simulink model "PFC_Plant_2022b_final"  (R2023b)
settings: Solver=FixedStepAuto  StartTime=0.0  StopTime=0.5  FixedStep=1e-5  RelTol=1e-3
undefined symbols (not defined in the file or in its folder): DiscIntNeverNeededParam
libraries: simulink x5, spsMeanLib x4, eeGeneralControl x2, eePowerMeasurement x1, spsTHDLib x1
settings Model: PacingRate=1000  Creator=tuca_v1  LastModifiedBy=Moisa Versatu
settings OptimizationCC: ReuseModelBlockBuffer=off
settings DebuggingCC: UnconnectedInputMsg=warning  UnconnectedOutputMsg=warning  UnconnectedLineMsg=warning
settings ModelReferenceCC: EnableRefExpFcnMdlSchedulingChecks=on
settings RTWCC: DLArmComputeVersion=19.05

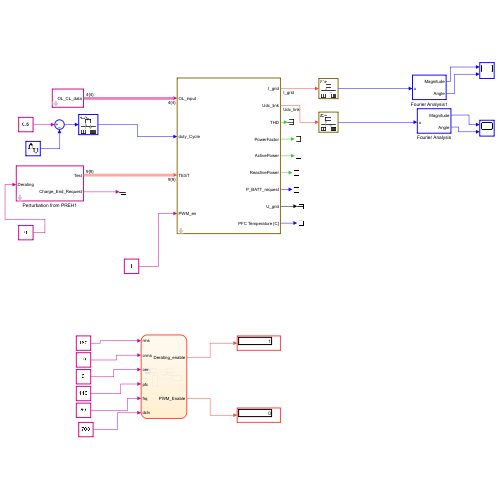
[thumbnail: Simulink's stored preview of the top-level diagram]
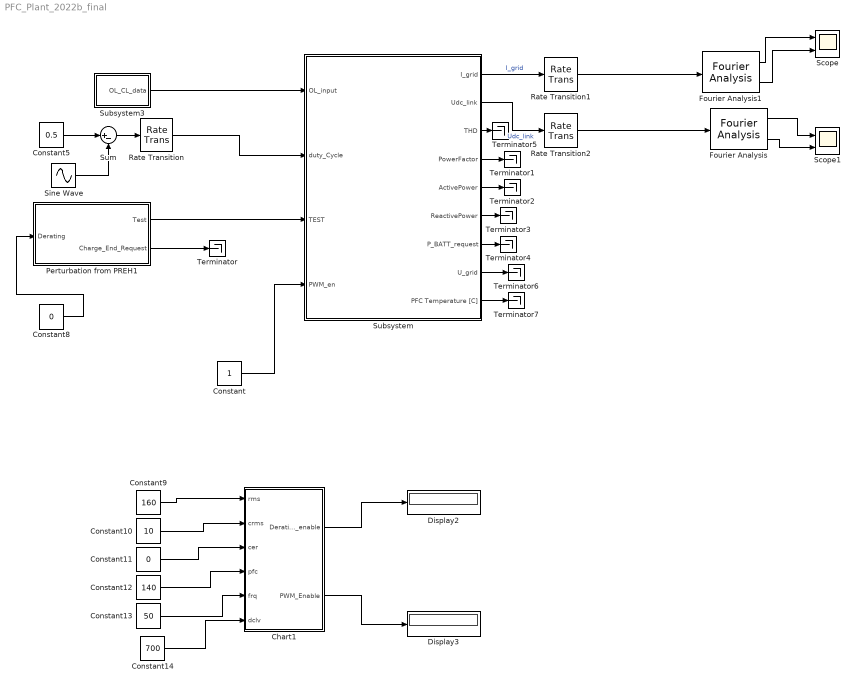
== system PFC_Plant_2022b_final ==
  Chart1 : Stateflow chart  TreatAsAtomicUnit=on
  Constant : Constant
  Constant10 : Constant  Value=10
  Constant11 : Constant  Value=0
  Constant12 : Constant  Value=140
  Constant13 : Constant  Value=50
  Constant14 : Constant  Value=700
  Constant5 : Constant  Value=0.5
  Constant8 : Constant  Value=0
  Constant9 : Constant  Value=160
  Display2 : Display
  Display3 : Display
  Fourier Analysis : eeGeneralControl/Fourier Analysis  f=50  n=[1]  M0=1  Ph0=0  BufferSize=8192  Ts=1e-4
      settings: LibrarySourceBlock=ee_sl_lib/General Control/Fourier Analysis
  Fourier Analysis1 : eeGeneralControl/Fourier Analysis  f=50  n=[1]  M0=1  Ph0=0  BufferSize=8192  Ts=1e-4
      settings: LibrarySourceBlock=ee_sl_lib/General Control/Fourier Analysis
  Perturbation from PREH1 : Subsystem  mask{Overwrite_power=0, Uin_rms=220, F_grid=50, RMS_variation=0, Freq_variation=0, AC_harmonics=0, Charge_End_Request=0, Coolant_mass_flow=0.1, Coolant_temperature=60}
      mask prompts: Charge_End_Request "Charge End Request"
  Rate Transition : RateTransition  OutPortSampleTime=1e-4
  Rate Transition1 : RateTransition  OutPortSampleTime=1e-4
  Rate Transition2 : RateTransition  OutPortSampleTime=1e-4
  Scope : Scope  NumInputPorts=2
  Scope1 : Scope  NumInputPorts=2
  Sine Wave : Sin  Amplitude=0.02  Frequency=2*pi*50  SampleTime=1e-4
  Subsystem : Subsystem  mask{f_grid=50}
      mask init:
      | Ts_thermal = 1e-2;
      | Tc = 1e-5;
  Subsystem3 : Subsystem  mask{DC_AC=0, Uin_rms_OL=220, UDC_link_OL=220, Power_out=0}
      mask prompts: DC_AC "DC_AC enum"
  Sum : Sum  Inputs=|+-
  Terminator{,1..7} (8 alike) : Terminator
  wires:
  Subsystem3/1(OL_CL_data) -> Subsystem/1(OL_input)
  Subsystem/8(U_grid) -> Terminator6/1
  Perturbation from PREH1/1(Test) -> Subsystem/3(TEST)
  Constant5/1 -> Sum/1
  Sine Wave/1 -> Sum/2
  Sum/1 -> Rate Transition/1
  Rate Transition/1 -> Subsystem/2(duty_Cycle)
  Subsystem/2(Udc_link) -> Rate Transition2/1  "Udc_link"
  Subsystem/1(I_grid) -> Rate Transition1/1  "I_grid"
  Rate Transition2/1 -> Fourier Analysis/1
  Constant/1 -> Subsystem/4(PWM_en)
  Constant8/1 -> Perturbation from PREH1/1(Derating)
  Perturbation from PREH1/2(Charge_End_Request) -> Terminator/1
  Subsystem/7(P_BATT_request) -> Terminator4/1
  Subsystem/6(ReactivePower) -> Terminator3/1
  Subsystem/5(ActivePower) -> Terminator2/1
  Subsystem/4(PowerFactor) -> Terminator1/1
  Subsystem/3(THD) -> Terminator5/1
  Subsystem/9(PFC Temperature [C]) -> Terminator7/1
  Rate Transition1/1 -> Fourier Analysis1/1
  Fourier Analysis/1 -> Scope1/1
  Fourier Analysis1/1 -> Scope/1
  Chart1/1(Derating_enable) -> Display2/1
  Constant11/1 -> Chart1/3(cer)
  Constant10/1 -> Chart1/2(crms)
  Constant9/1 -> Chart1/1(rms)
  Constant13/1 -> Chart1/5(frq)
  Constant14/1 -> Chart1/6(dclv)
  Constant12/1 -> Chart1/4(pfc)
  Chart1/2(PWM_Enable) -> Display3/1
  Fourier Analysis1/2 -> Scope/2
  Fourier Analysis/2 -> Scope1/2

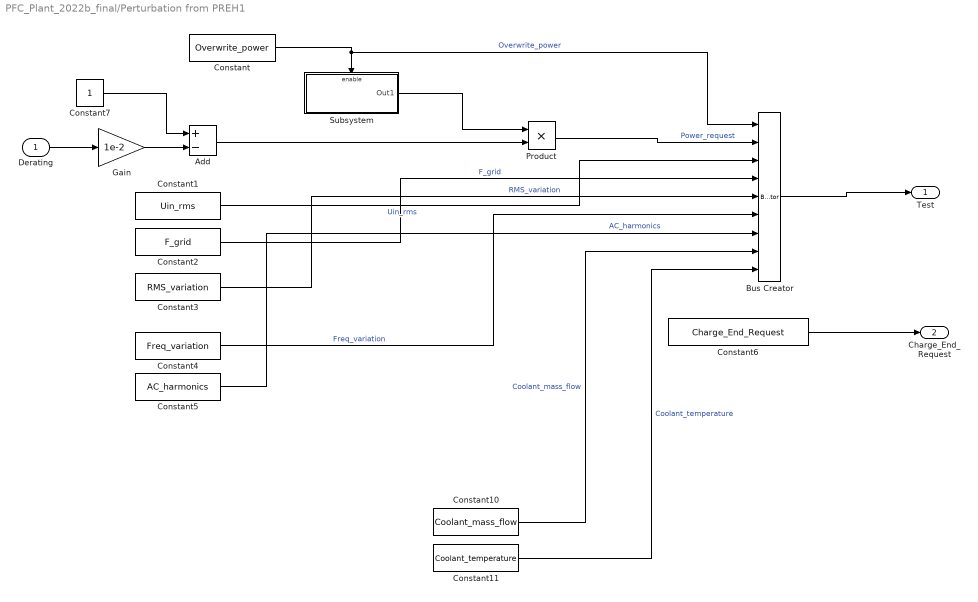
== system PFC_Plant_2022b_final/Perturbation from PREH1 ==
  Derating : Inport
  Add : Sum  Inputs=+-
  Bus Creator : BusCreator  Inputs=9
  Constant : Constant  Value=Overwrite_power
  Constant1 : Constant  Value=Uin_rms
  Constant10 : Constant  Value=Coolant_mass_flow
  Constant11 : Constant  Value=Coolant_temperature
  Constant2 : Constant  Value=F_grid
  Constant3 : Constant  Value=RMS_variation
  Constant4 : Constant  Value=Freq_variation
  Constant5 : Constant  Value=AC_harmonics
  Constant6 : Constant  Value=Charge_End_Request
  Constant7 : Constant
  Gain : Gain  Gain=1e-2
  Product : Product
  Subsystem : Subsystem
  Test : Outport
  Charge_End_Request : Outport  Port=2
  wires:
  Constant/1 -> Bus Creator/1, Subsystem/Enable  "Overwrite_power"
  Bus Creator/1 -> Test/1
  Subsystem/1(Out1) -> Product/1
  Constant1/1 -> Bus Creator/3  "Uin_rms"
  Constant2/1 -> Bus Creator/4  "F_grid"
  Constant3/1 -> Bus Creator/5  "RMS_variation"
  Constant4/1 -> Bus Creator/6  "Freq_variation"
  Constant5/1 -> Bus Creator/7  "AC_harmonics"
  Add/1 -> Product/2
  Product/1 -> Bus Creator/2  "Power_request"
  Constant6/1 -> Charge_End_Request/1
  Gain/1 -> Add/2
  Derating/1 -> Gain/1
  Constant7/1 -> Add/1
  Constant10/1 -> Bus Creator/8  "Coolant_mass_flow"
  Constant11/1 -> Bus Creator/9  "Coolant_temperature"

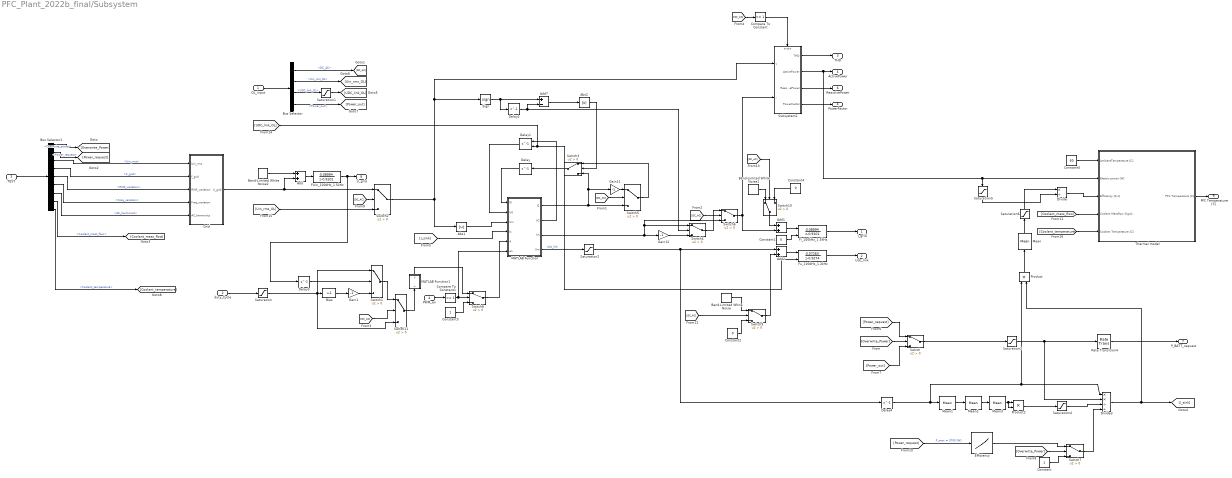
== system PFC_Plant_2022b_final/Subsystem ==
  OL_input : Inport
  duty_Cycle : Inport  Port=2
  TEST : Inport  Port=3
  PWM_en : Inport  Port=4
  Abs1 : Abs  SaturateOnIntegerOverflow=off
  Abs2 : Abs  SaturateOnIntegerOverflow=off
  Add : Sum
  Add1 : Sum
  Add2 : Sum
  Add7 : Sum  Inputs=+-
  Band-Limited White Noise : simulink/Sources/Band-Limited White Noise  Cov=5e-7  Ts=1e-5  seed=[23341]
  Band-Limited White Noise1 : simulink/Sources/Band-Limited White Noise  Cov=5e-9  Ts=1e-5  seed=[23342]
  Band-Limited White Noise2 : simulink/Sources/Band-Limited White Noise  Cov=5e-7  Ts=1e-5  seed=[23342]
  Bias : Bias  Bias=-1  SaturateOnIntegerOverflow=off
  Bus Selector : BusSelector  OutputSignals=DC_AC,Uin_rms_OL,UDC_link_OL,Power_out
  Bus Selector1 : BusSelector  OutputSignals=Overwrite_power,Power_request,Uin_rms,F_grid,RMS_variation,Freq_variation,AC_harmonics,Coolant_mass_flow,Coolant_temperature
  Compare To Constant : simulink/Logic and Bit Operations/Compare To Constant  relop===  const=1  OutDataTypeStr=boolean
  Compare To Constant1 : simulink/Logic and Bit Operations/Compare To Constant  relop===  const=1  OutDataTypeStr=boolean
  Constant : Constant
  Constant1 : Constant  Value=0
  Constant2 : Constant  Value=0
  Constant3 : Constant
  Constant4 : Constant  Value=0
  Constant5 : Constant  Value=60
  Delay : Delay  DelayLength=1  SampleTime=1e-5
  Delay1 : Delay  DelayLength=1  InitialConditionSource=Input port  SampleTime=1e-5
      settings: InputPortMap=u0,p4
  Delay2 : Delay  DelayLength=1  SampleTime=1e-5
  Delay3 : Delay  DelayLength=1  SampleTime=Tc
  Delay4 : Delay  DelayLength=1  SampleTime=Tc
  Divide : Product  Inputs=*/
  Divide3 : Product  Inputs=**//
  Efficiency : Lookup_n-D  NumberOfTableDimensions=1  BreakpointsForDimension1=[500 1000 1500 2000 2500 3000 3500 5000 7000 9000 11100]/3  Table="[0.85 0.92 0.95  0.97  0.975 0.97 0.967 0.963 0.96 0.959 0.955]"  ExtrapMethod=Clip  UseLastTableValue=on  InternalRulePriority=Speed  RndMeth=Simplest
  FUin_100kHz_1.5kHz : DiscreteTransferFcn  Numerator=[0.08994]  Denominator=[1 -0.9101]  SampleTime=Tc
  Fi_100kHz_1.5kHz : DiscreteTransferFcn  Numerator=[0.08994]  Denominator=[1 -0.9101]  InitialStatesSource=Input port  SampleTime=Tc
      settings: InputPortMap=u0,p5
  Fu_100kHz_1.2kHz : DiscreteTransferFcn  Numerator=[0.07263]  Denominator=[1 -0.9274]  InitialStatesSource=Input port  SampleTime=Tc
      settings: InputPortMap=u0,p5
  Gain1 : Gain  Gain=-1
  Gain11 : Gain  Gain=-1
  Gain12 : Gain  Gain=-1
  Grid : Subsystem
  MATLAB Function : MATLAB Function  TreatAsAtomicUnit=on
  MATLAB Function1 : MATLAB Function  TreatAsAtomicUnit=on
  Mean : spsMeanLib/Mean  Freq=5  Vinit=0  Ts=Tc
  Mean1 : spsMeanLib/Mean  Freq=2*f_grid  Vinit=0  Ts=Tc
  Mean2 : spsMeanLib/Mean  Freq=2*f_grid  Vinit=0  Ts=Tc
  Mean3 : spsMeanLib/Mean  Freq=2*f_grid  Vinit=0  Ts=Tc
  Product : Product
  Product2 : Product
  Rate Transition4 : RateTransition  OutPortSampleTime=1e-2
  Saturation : Saturate  UpperLimit=0.998  LowerLimit=0.002
  Saturation1 : Saturate  UpperLimit=inf  LowerLimit=1e-4
  Saturation2 : Saturate  UpperLimit=inf  LowerLimit=1e-4
  Saturation3 : Saturate  UpperLimit=1e3  LowerLimit=0
  Saturation4 : Saturate  UpperLimit=inf  LowerLimit=1e-4
  Saturation5 : Saturate  UpperLimit=1e4  LowerLimit=1
  Saturation6 : Saturate  UpperLimit=1e4  LowerLimit=1
  Sign : Signum
  Subsystem1 : Subsystem
  Switch{,1..11} (12 alike) : Switch  Criteria=u2 > Threshold  SaturateOnIntegerOverflow=off  InputSameDT=off
  Thermal model : Subsystem
  I_grid : Outport
  Udc_link : Outport  Port=2
  THD : Outport  Port=3
  PowerFactor : Outport  Port=4
  ActivePower : Outport  Port=5
  ReactivePower : Outport  Port=6
  P_BATT_request : Outport  Port=7
  U_grid : Outport  Port=8
  PFC Temperature [C] : Outport  Port=9
  wires:
  MATLAB Function/1(I2) -> Switch3/3, Gain11/1, Switch5/3
  Gain12/1 -> Switch4/3
  [UDC_link_OL] -> Delay1/2, Fu_100kHz_1.2kHz/2
  [I_sink] -> MATLAB Function/4(Is)
  Abs2/1 -> Switch3/2
  Add7/1 -> Abs2/1
  Delay1/1 -> MATLAB Function/2(U0)
  Switch3/1 -> Delay/1
  Abs1/1 -> MATLAB Function/3(Uin)
  duty_Cycle/1 -> Saturation/1
  Sign/1 -> Delay2/1, Add7/1
  Switch5/1 -> Switch3/1
  Delay2/1 -> Switch4/2, Add7/2
  MATLAB Function/2(U2) -> Delay1/1
  MATLAB Function/3(Im) -> Gain12/1, Switch4/1, Switch6/3
  Switch6/1 -> Subsystem1/2(i), Add1/2
  Saturation/1 -> Switch11/3, Switch1/1, Bias/1
  Bias/1 -> Gain1/1
  Add1/1 -> Fi_100kHz_1.5kHz/1
  Add2/1 -> Fu_100kHz_1.2kHz/1
  Band-Limited White Noise1/1 -> Switch10/1
  Fi_100kHz_1.5kHz/1 -> I_grid/1
  Fu_100kHz_1.2kHz/1 -> Udc_link/1
  Switch2/1 -> Subsystem1/1(v), Sign/1, Abs1/1
  [Uin_rms_OL] -> Switch2/3
  Gain11/1 -> Switch5/1
  [DC_AC] -> Switch5/2
  [DC_AC] -> Switch6/2
  Switch4/1 -> Switch6/1
  Subsystem1/1(THD) -> THD/1
  Subsystem1/2(ActivePower) -> Thermal model/2(Electric power [W]), Saturation5/1, ActivePower/1
  Subsystem1/3(ReactivePower) -> ReactivePower/1
  Subsystem1/4(PowerFactor) -> PowerFactor/1
  [DC_AC] -> Compare To Constant/1
  Constant1/1 -> Fi_100kHz_1.5kHz/2
  TEST/1 -> Bus Selector1/1
  Switch/1 -> Saturation3/1
  MATLAB Function/4(Um) -> Saturation2/1  "Udc_link"
  Mean1/1 -> Mean2/1
  Rate Transition4/1 -> P_BATT_request/1
  Mean2/1 -> Mean3/1
  Band-Limited White Noise/1 -> Switch9/1
  Switch10/1 -> Add1/1
  [DC_AC] -> Switch2/2
  Mean3/1 -> Product2/2, Product2/1
  Product2/1 -> Saturation4/1
  Saturation3/1 -> Divide3/2, Rate Transition4/1
  Delay4/1 -> Divide3/1, Product/1, Mean1/1
  Compare To Constant/1 -> Subsystem1/Enable
  OL_input/1 -> Bus Selector/1
  Bus Selector/1 -> [DC_AC]  "<DC_AC>"
  Bus Selector/2 -> [Uin_rms_OL]  "<Uin_rms_OL>"
  Bus Selector/3 -> Saturation1/1  "<UDC_link_OL>"
  [DC_AC] -> Switch9/2
  Switch9/1 -> Add2/2
  Constant2/1 -> Switch9/3
  [DC_AC] -> Switch10/2
  Constant4/1 -> Switch10/3
  Grid/1(U_grid) -> Switch2/1, Add/2
  Gain1/1 -> Switch1/3
  Switch11/1 -> MATLAB Function1/1(u)
  Delay3/1 -> Switch1/2
  FUin_100kHz_1.5kHz/1 -> Delay3/1, U_grid/1
  Add/1 -> FUin_100kHz_1.5kHz/1
  Band-Limited White Noise2/1 -> Add/1
  Divide3/1 -> [I_sink], Product/2
  Switch8/1 -> MATLAB Function/5(d)
  Switch1/1 -> Switch11/1
  [DC_AC] -> Switch11/2
  Bus Selector1/1 -> [Overwrite_Power]  "<Overwrite_power>"
  [Overwrite_Power] -> Switch/2
  Bus Selector1/2 -> [Power_request]  "<Power_request>"
  [Power_request] -> Switch/1
  Bus Selector/4 -> [Power_out]  "<Power_out>"
  [Power_out] -> Switch/3
  Switch7/1 -> Divide3/4
  [Overwrite_Power] -> Switch7/2
  Efficiency/1 -> Switch7/1
  Constant/1 -> Switch7/3
  [Power_request] -> Efficiency/1  "P_max = 3700 [W]"
  Bus Selector1/3 -> Grid/1(Uin_rms)  "<Uin_rms>"
  Bus Selector1/4 -> Grid/2(f_grid)  "<F_grid>"
  Bus Selector1/5 -> Grid/3(RMS_variation)  "<RMS_variation>"
  Bus Selector1/6 -> Grid/4(Freq_variation)  "<Freq_variation>"
  Bus Selector1/7 -> Grid/5(AC_harmonics)  "<AC_harmonics>"
  Saturation2/1 -> Add2/1, Delay4/1
  Saturation1/1 -> [UDC_link_OL]
  Saturation4/1 -> Divide3/3
  PWM_en/1 -> Compare To Constant1/1
  Compare To Constant1/1 -> Switch8/2, MATLAB Function/6(en)
  MATLAB Function1/1(y) -> Switch8/1
  Constant3/1 -> Switch8/3
  Delay/1 -> MATLAB Function/1(I0)
  Product/1 -> Mean/1
  Mean/1 -> Saturation6/1
  Divide/1 -> Thermal model/3(Efficiency [0-1])
  Constant5/1 -> Thermal model/1(AmbientTemperature [C])
  [Coolant_temperature] -> Thermal model/5(Coolant Temperature [C])
  [Coolant_mass_flow] -> Thermal model/4(Coolant Massflow [kg/s])
  Thermal model/1(PFC Temperature [C]) -> PFC Temperature [C]/1
  Saturation5/1 -> Divide/2
  Saturation6/1 -> Divide/1
  Bus Selector1/8 -> [Coolant_mass_flow]  "<Coolant_mass_flow>"
  Bus Selector1/9 -> [Coolant_temperature]  "<Coolant_temperature>"

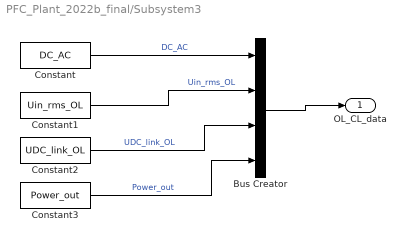
== system PFC_Plant_2022b_final/Subsystem3 ==
  Bus Creator : BusCreator  Inputs=4
  Constant : Constant  Value=DC_AC
  Constant1 : Constant  Value=Uin_rms_OL
  Constant2 : Constant  Value=UDC_link_OL
  Constant3 : Constant  Value=Power_out
  OL_CL_data : Outport
  wires:
  Bus Creator/1 -> OL_CL_data/1
  Constant/1 -> Bus Creator/1  "DC_AC"
  Constant1/1 -> Bus Creator/2  "Uin_rms_OL"
  Constant2/1 -> Bus Creator/3  "UDC_link_OL"
  Constant3/1 -> Bus Creator/4  "Power_out"

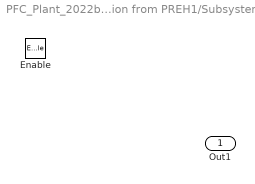
== system PFC_Plant_2022b_final/Perturbation from PREH1/Subsystem ==
  Enable : EnablePort
  Out1 : Outport

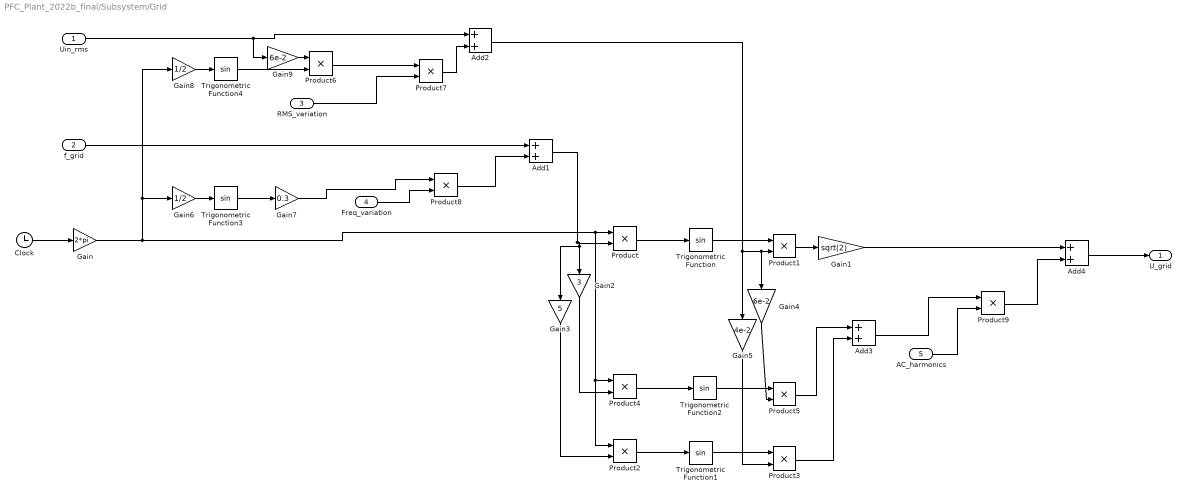
== system PFC_Plant_2022b_final/Subsystem/Grid ==
  Uin_rms : Inport
  f_grid : Inport  Port=2
  RMS_variation : Inport  Port=3
  Freq_variation : Inport  Port=4
  AC_harmonics : Inport  Port=5
  Add1 : Sum
  Add2 : Sum
  Add3 : Sum  Inputs=2
  Add4 : Sum  Inputs=2
  Clock : Clock
  Gain : Gain  Gain=2*pi
  Gain1 : Gain  Gain=sqrt(2)
  Gain2 : Gain  Gain=3
  Gain3 : Gain  Gain=5
  Gain4 : Gain  Gain=6e-2
  Gain5 : Gain  Gain=4e-2
  Gain6 : Gain  Gain=1/2
  Gain7 : Gain  Gain=0.3
  Gain8 : Gain  Gain=1/2
  Gain9 : Gain  Gain=6e-2
  Product{,1..9} (10 alike) : Product
  Trigonometric Function{,1..4} (5 alike) : Trigonometry
  U_grid : Outport
  wires:
  Clock/1 -> Gain/1
  Gain/1 -> Gain8/1, Gain6/1, Product4/1, Product2/1, Product/1
  Product/1 -> Trigonometric Function/1
  Trigonometric Function/1 -> Product1/1
  Product1/1 -> Gain1/1
  Gain1/1 -> Add4/1
  Add1/1 -> Gain3/1, Gain2/1, Product/2
  Product2/1 -> Trigonometric Function1/1
  Trigonometric Function1/1 -> Product3/1
  Add2/1 -> Gain5/1, Gain4/1, Product1/2
  Product3/1 -> Add3/2
  Add4/1 -> U_grid/1
  Trigonometric Function2/1 -> Product5/1
  Product4/1 -> Trigonometric Function2/1
  Product5/1 -> Add3/1
  Gain2/1 -> Product4/2
  Gain3/1 -> Product2/2
  Gain4/1 -> Product5/2
  Gain5/1 -> Product3/2
  f_grid/1 -> Add1/1
  Trigonometric Function3/1 -> Gain7/1
  Gain6/1 -> Trigonometric Function3/1
  Gain7/1 -> Product8/1
  Uin_rms/1 -> Gain9/1, Add2/1
  Gain8/1 -> Trigonometric Function4/1
  Trigonometric Function4/1 -> Product6/2
  Product6/1 -> Product7/1
  Gain9/1 -> Product6/1
  Product7/1 -> Add2/2
  Product8/1 -> Add1/2
  Add3/1 -> Product9/1
  Product9/1 -> Add4/2
  RMS_variation/1 -> Product7/2
  Freq_variation/1 -> Product8/2
  AC_harmonics/1 -> Product9/2

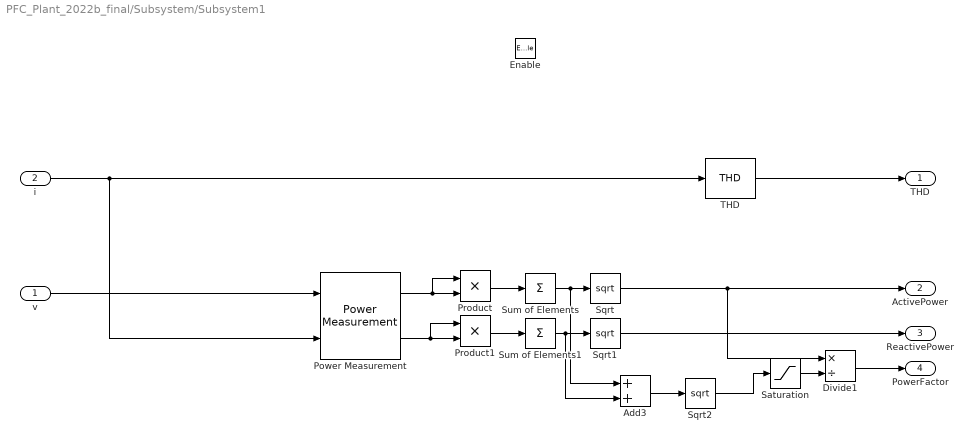
== system PFC_Plant_2022b_final/Subsystem/Subsystem1 ==
  v : Inport
  i : Inport  Port=2
  Enable : EnablePort
  Add3 : Sum
  Divide1 : Product  Inputs=*/
  Power Measurement : eePowerMeasurement/Power Measurement  LabelModeActiveChoice=Discrete  F=f_grid  K=[0 1 2 3 5 7 9 11 13]  Ts=1/2e4
  Product : Product
  Product1 : Product
  Saturation : Saturate  UpperLimit=inf  LowerLimit=1e-4
  Sqrt : Sqrt
  Sqrt1 : Sqrt
  Sqrt2 : Sqrt
  Sum of Elements : Sum  Inputs=+
  Sum of Elements1 : Sum  Inputs=+
  "THD " : spsTHDLib/THD  Freq=f_grid  Ts=1/2e4
  THD : Outport
  ActivePower : Outport  Port=2
  ReactivePower : Outport  Port=3
  PowerFactor : Outport  Port=4
  wires:
  Sqrt/1 -> ActivePower/1, Divide1/1
  Add3/1 -> Sqrt2/1
  Power Measurement/2 -> Product1/1, Product1/2
  "THD "/1 -> THD/1
  Power Measurement/1 -> Product/1, Product/2
  Sum of Elements1/1 -> Add3/2, Sqrt1/1
  Product/1 -> Sum of Elements/1
  i/1 -> Power Measurement/2, "THD "/1
  Sqrt2/1 -> Saturation/1
  Product1/1 -> Sum of Elements1/1
  Sum of Elements/1 -> Add3/1, Sqrt/1
  Sqrt1/1 -> ReactivePower/1
  Divide1/1 -> PowerFactor/1
  v/1 -> Power Measurement/1
  Saturation/1 -> Divide1/2

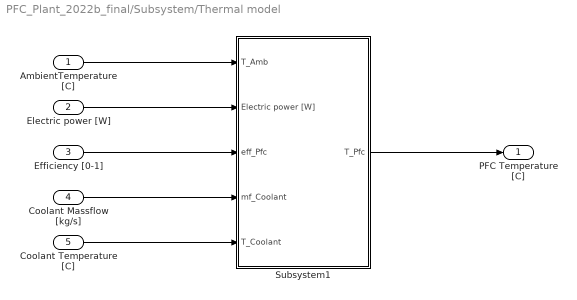
== system PFC_Plant_2022b_final/Subsystem/Thermal model ==
  AmbientTemperature [C] : Inport
  Electric power [W] : Inport  Port=2
  Efficiency [0-1] : Inport  Port=3
  Coolant Massflow [kg/s] : Inport  Port=4
  Coolant Temperature [C] : Inport  Port=5
  Subsystem1 : Subsystem
  PFC Temperature [C] : Outport
  wires:
  Subsystem1/1(T_Pfc) -> PFC Temperature [C]/1
  AmbientTemperature [C]/1 -> Subsystem1/1(T_Amb)
  Coolant Massflow [kg/s]/1 -> Subsystem1/4(mf_Coolant)
  Coolant Temperature [C]/1 -> Subsystem1/5(T_Coolant)
  Electric power [W]/1 -> Subsystem1/2(Electric power [W])
  Efficiency [0-1]/1 -> Subsystem1/3(eff_Pfc)

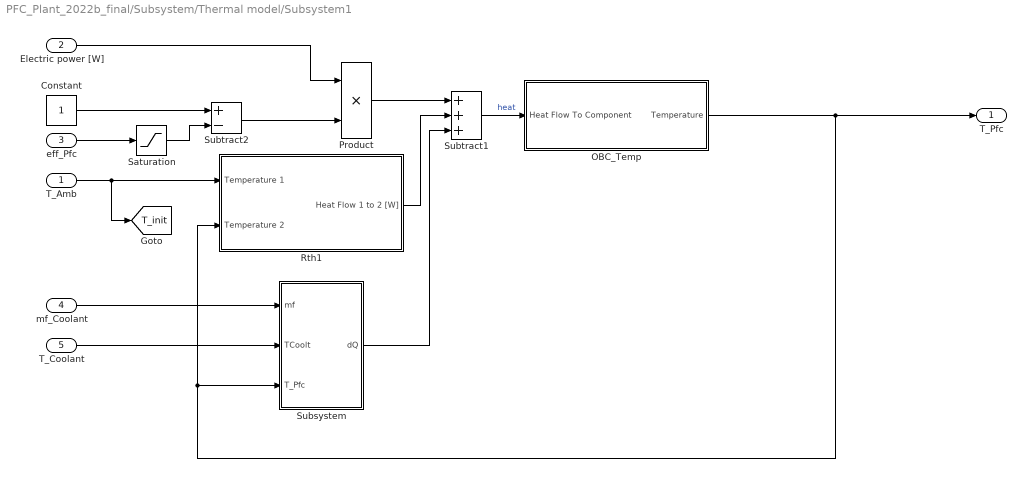
== system PFC_Plant_2022b_final/Subsystem/Thermal model/Subsystem1 ==
  T_Amb : Inport
  Electric power [W] : Inport  Port=2
  eff_Pfc : Inport  Port=3
  mf_Coolant : Inport  Port=4
  T_Coolant : Inport  Port=5
  Constant : Constant
  OBC_Temp : Subsystem
  Product : Product
  Rth1 : Subsystem
  Saturation : Saturate  UpperLimit=1  LowerLimit=0
  Subsystem : Subsystem
  Subtract1 : Sum  Inputs=+++
  Subtract2 : Sum  Inputs=+-
  T_Pfc : Outport
  tag scope: T_init=global
  wires:
  Subtract1/1 -> OBC_Temp/1(Heat Flow To Component)  "heat"
  Product/1 -> Subtract1/1
  T_Amb/1 -> Rth1/1(Temperature 1), [T_init]
  Rth1/1(Heat Flow 1 to 2 [W]) -> Subtract1/2
  Constant/1 -> Subtract2/1
  Electric power [W]/1 -> Product/1
  Subsystem/1(dQ) -> Subtract1/3
  mf_Coolant/1 -> Subsystem/1(mf)
  T_Coolant/1 -> Subsystem/2(TCoolt)
  Subtract2/1 -> Product/2
  eff_Pfc/1 -> Saturation/1
  Saturation/1 -> Subtract2/2
  OBC_Temp/1(Temperature) -> T_Pfc/1, Subsystem/3(T_Pfc), Rth1/2(Temperature 2)

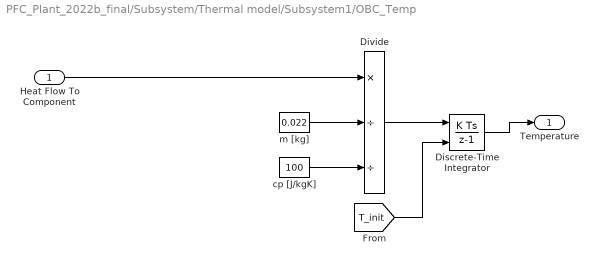
== system PFC_Plant_2022b_final/Subsystem/Thermal model/Subsystem1/OBC_Temp ==
  Heat Flow To Component : Inport
  Discrete-Time Integrator : DiscreteIntegrator  InitialConditionSource=external  InitialCondition=23  SampleTime=Ts_thermal  ICPrevOutput=DiscIntNeverNeededParam  ICPrevScaledInput=DiscIntNeverNeededParam
  Divide : Product  Inputs=*//
  cp [J/kgK] : Constant  Value=100
  m [kg] : Constant  Value=0.022
  Temperature : Outport
  wires:
  cp [J/kgK]/1 -> Divide/3
  m [kg]/1 -> Divide/2
  Heat Flow To Component/1 -> Divide/1
  Divide/1 -> Discrete-Time Integrator/1
  Discrete-Time Integrator/1 -> Temperature/1
  [T_init] -> Discrete-Time Integrator/2

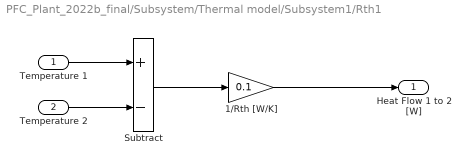
== system PFC_Plant_2022b_final/Subsystem/Thermal model/Subsystem1/Rth1 ==
  Temperature 1 : Inport
  Temperature 2 : Inport  Port=2
  1/Rth [W/K] : Gain  Gain=0.1
  Subtract : Sum  Inputs=+-
  Heat Flow 1 to 2 [W] : Outport
  wires:
  1/Rth [W/K]/1 -> Heat Flow 1 to 2 [W]/1
  Subtract/1 -> 1/Rth [W/K]/1
  Temperature 1/1 -> Subtract/1
  Temperature 2/1 -> Subtract/2

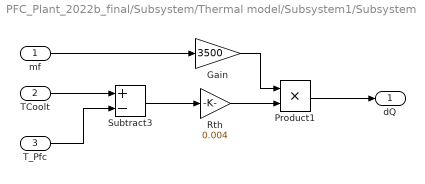
== system PFC_Plant_2022b_final/Subsystem/Thermal model/Subsystem1/Subsystem ==
  mf : Inport
  TCoolt : Inport  Port=2
  T_Pfc : Inport  Port=3
  Gain : Gain  Gain=3500
  Product1 : Product
  Rth : Gain  Gain=0.004
  Subtract3 : Sum  Inputs=+-
  dQ : Outport
  wires:
  TCoolt/1 -> Subtract3/1
  Subtract3/1 -> Rth/1
  Gain/1 -> Product1/1
  Product1/1 -> dQ/1
  T_Pfc/1 -> Subtract3/2
  Rth/1 -> Product1/2
  mf/1 -> Gain/1

== matlab function PFC_Plant_2022b_final/Subsystem/MATLAB Function1 ==
  data: u input; y output
function y = fcn(u)

y = round(u/0.2e-2)*0.2e-2;

== matlab function PFC_Plant_2022b_final/Subsystem/MATLAB Function ==
  data: I0 input; I2 output; U0 input; Uin input; Is input; d input; U2 output; Im output; Um output; en input
function [I2 , U2 , Im , Um] = fcn(I0 , U0 , Uin , Is , d, en)
tsw = 1e-5;
vct = [Uin ; Is ; I0 ; U0];
t = d*tsw;
% fon = real([[                                                                                -(10^(1/2)*17^(1/2)*exp(-(428161227780181248*t)/2568967366681087)*sinh((10^(1/2)*17^(1/2)*t*109688310119566390625i)/918734323983581184)*72057594037927936i)/877506480956531125,                                                                                                                                                                                     1 - exp(-(428161227780181248*t)/2568967366681087)*cosh((10^(1/2)*17^(1/2)*t*109688310119566390625i)/918734323983581184), exp(-(428161227780181248*t)/2568967366681087)*(cosh((10^(1/2)*17^(1/2)*t*109688310119566390625i)/918734323983581184) + (10^(1/2)*17^(1/2)*sinh((10^(1/2)*17^(1/2)*t*109688310119566390625i)/918734323983581184)*125437859701224975i)/15275632820491293824),                                                                              (10^(1/2)*17^(1/2)*exp(-(428161227780181248*t)/2568967366681087)*sinh((10^(1/2)*17^(1/2)*t*109688310119566390625i)/918734323983581184)*72057594037927936i)/877506480956531125] ; ...
%             [1 - exp(-(428161227780181248*t)/2568967366681087)*(cosh((10^(1/2)*17^(1/2)*t*109688310119566390625i)/918734323983581184) - (10^(1/2)*17^(1/2)*sinh((10^(1/2)*17^(1/2)*t*109688310119566390625i)/918734323983581184)*125437859701224975i)/15275632820491293824), (6165521680034609*exp(-(428161227780181248*t)/2568967366681087)*(cosh((10^(1/2)*17^(1/2)*t*109688310119566390625i)/918734323983581184) + (sinh((10^(1/2)*17^(1/2)*t*109688310119566390625i)/918734323983581184)*9227758726500357743883612110375i)/987984465162757204733090332672))/61655216800346088 - 1/10,                                                                                   -(170^(1/2)*exp(-(428161227780181248*t)/2568967366681087)*sinh((10^(1/2)*17^(1/2)*t*109688310119566390625i)/918734323983581184)*216172782113783808i)/2983522035252205825, exp(-(428161227780181248*t)/2568967366681087)*(cosh((10^(1/2)*17^(1/2)*t*109688310119566390625i)/918734323983581184) - (10^(1/2)*17^(1/2)*sinh((10^(1/2)*17^(1/2)*t*109688310119566390625i)/918734323983581184)*125437859701224975i)/15275632820491293824)]]);
fon = real([[                                                                                -(10^(1/2)*17^(1/2)*exp(-(428161227780181248*t)/2568967366681087)*sinh((10^(1/2)*17^(1/2)*t*109688310119566390625i)/918734323983581184)*72057594037927936i)/877506480956531125,                                                                                                                                                                                     1 - exp(-(428161227780181248*t)/2568967366681087)*cosh((10^(1/2)*17^(1/2)*t*109688310119566390625i)/918734323983581184), exp(-(428161227780181248*t)/2568967366681087)*(cosh((10^(1/2)*17^(1/2)*t*109688310119566390625i)/918734323983581184) + (10^(1/2)*17^(1/2)*sinh((10^(1/2)*17^(1/2)*t*109688310119566390625i)/918734323983581184)*125437859701224975i)/15275632820491293824),                                                                              (10^(1/2)*17^(1/2)*exp(-(428161227780181248*t)/2568967366681087)*sinh((10^(1/2)*17^(1/2)*t*109688310119566390625i)/918734323983581184)*72057594037927936i)/877506480956531125] ; ...
            [1 - exp(-(428161227780181248*t)/2568967366681087)*(cosh((10^(1/2)*17^(1/2)*t*109688310119566390625i)/918734323983581184) - (10^(1/2)*17^(1/2)*sinh((10^(1/2)*17^(1/2)*t*109688310119566390625i)/918734323983581184)*125437859701224975i)/15275632820491293824), (6165521680034609*exp(-(428161227780181248*t)/2568967366681087)*(cosh((10^(1/2)*17^(1/2)*t*109688310119566390625i)/918734323983581184) + (sinh((10^(1/2)*17^(1/2)*t*109688310119566390625i)/918734323983581184)*9227758726500357743883612110375i)/987984465162757204733090332672))/61655216800346088 - 1/10,                                                                                   -(170^(1/2)*exp(-(428161227780181248*t)/2568967366681087)*sinh((10^(1/2)*17^(1/2)*t*109688310119566390625i)/918734323983581184)*216172782113783808i)/2983522035252205825, exp(-(428161227780181248*t)/2568967366681087)*(cosh((10^(1/2)*17^(1/2)*t*109688310119566390625i)/918734323983581184) - (10^(1/2)*17^(1/2)*sinh((10^(1/2)*17^(1/2)*t*109688310119566390625i)/918734323983581184)*125437859701224975i)/15275632820491293824)]]);
t = (1-d)*tsw;

% foff = [[10 - 10*exp(-(500*t)/3),             0, exp(-(500*t)/3), 0]; ...
%         [                      0, -(50000*t)/41,               0, 1]];

foff = [[10 - 10*exp(-(500*t)/3),             0, exp(-(500*t)/3), 0] ; ...
        [                      0, -(25000*t)/17,               0, 1]];
ON_end = fon*vct;
if en == 0

    ON_end(1) = max(0,ON_end(1));
end

OFF_end = foff*[Uin ; Is ;ON_end];
if en == 0

    OFF_end(1) = max(0,OFF_end(1));
end
I2 = OFF_end(1);
U2 = OFF_end(2);

MEAN = ([I0 ; U0] + ON_end)*d/2+(ON_end+[I2 ; U2])*(1-d)/2;
Im = MEAN(1);
Um = MEAN(2);

end

== stateflow chart PFC_Plant_2022b_final/Chart1 ==
  state Idle
    entry:
    flag1 = f(rms,frq,cer,pfc,crms);
    flag = f1(rms,frq,dclv,pfc,crms);
    during:
    if pfc>120
    Derating_enable=1;
    end
    flag1 = f(rms,frq,cer,pfc,crms);
    flag = f1(rms,frq,dclv,pfc,crms);
  state Pre_charge
    entry:
    flag1 = f(rms,frq,cer,pfc,crms);
    flag = f1(rms,frq,dclv,pfc,crms);
    during:
    if pfc>120
    Derating_enable=1;
    end
    flag1 = f(rms,frq,cer,pfc,crms);
  state Error
    entry:
    if flag==2
    fprintf('AC Undervoltage')
    end
    if flag==3
    fprintf('AC Overvoltage')
    end
    if flag==4
    fprintf('Underfrequency')
    end
    if flag==5
    fprintf('Overfrequency')
    end
    if flag==6
    fprintf('DC Link Undervoltage')
    end
    if flag==7
    fprintf('DC Link Overvoltage')
    end
    if flag==8
    fprintf('PFC Overheated')
    end
    if flag==9
    fprintf('AC Overcurrent')
    end
    during:
    flag = f1(rms,frq,dclv,pfc,crms)
  state Charging
    entry:
    flag = f(rms,frq,cer,pfc,crms);
    flag1 = f1(rms,frq,dclv,pfc,crms);
    during:
    if pfc>120
    Derating_enable=1;
    end
    flag = f(rms,frq,cer,pfc,crms);
    flag1 = f1(rms,frq,dclv,pfc,crms);
  (default) -> Idle
  Idle -> Pre_charge [order 1] : [flag1==1 && dclv<=400 ]
  Charging -> Idle [order 2] : [cer==1]
  Pre_charge -> Error [order 2] : [flag==0]
  Pre_charge -> Charging [order 1] : [flag1==1 && dclv>=600 && dclv<=800 && after(2,sec)]{PWM_Enable=1}
  Error -> Idle : [after(2,sec)]
  Idle -> Error [order 3] : [flag==0]
  Idle -> Charging [order 2] : [flag1==1 && dclv>=600 && dclv<=800]{PWM_Enable=1}
  Charging -> Error [order 1] : [flag==0]
  data: rms function_input; frq function_input; cer function_input; pfc function_input; crms function_input; flag1 function_output; rms function_input; frq function_input; dclv function_input; pfc function_input; crms function_input; flag function_output; Derating_enable output; rms input; crms input; cer input; pfc input; frq input; PWM_Enable output; dclv input; flag1 local; flag local
  function flag1 = f(rms,frq,cer,pfc,crms):
    | function flag1 = f(rms,frq,cer,pfc,crms)
    | flag1=1;
    | if rms<185 || rms>265
    |     flag1=0;
    | end
    | if frq<45 || frq>65
    |     flag1=0;
    | end
    | if cer~=0
    |     flag1=0;
    | end
    | if pfc>150
    |     flag1=0;
    | end
    | if crms>16
    |     flag1=0;
    | end
    | end
  function flag = f1(rms,frq,dclv,pfc,crms):
    | function flag = f1(rms,frq,dclv,pfc,crms)
    | flag=0;
    | if rms<185
    |     flag=2;
    | end
    | if rms>265
    |     flag=3;
    | end
    | if frq<45
    |     flag=4;
    | end
    | if frq>65
    |     flag=5;
    | end
    | if dclv<600
    |     flag=6;
    | end
    | if dclv>800
    |     flag=7;
    | end
    | if pfc>150
    |     flag=8;
    | end
    | if crms>16
    |     flag=9;
    | end
    | end
